simulink model "Galvo_sys_v20_scope"  (R2014a)
settings: Solver=ode45  StartTime=0.0  StopTime=5e-3  MaxStep=1e-4  RelTol=1e-3
InitFcn:
  | Kp_cc = evalin('base','Kp_cc');
  | init = evalin('base','init');
StartFcn:
  | Kp_cc = evalin('base','Kp_cc')
model workspace (MATLAB code in the model file):
  | Kp_cc = evalin('base','Kp_cc');
libraries: simulink x2
settings Model: Kp_cc=1  BufferReuse=off  Creator=mainster  LastModifiedBy=mainster
settings DataIOCC: SaveFormat=StructureWithTime
settings OptimizationCC: BlockReduction=off  InlineParams=on  OptimizeBlockIOStorage=off  BufferReuse=off  GlobalBufferReuse=off  ExpressionFolding=off  LocalBlockOutputs=off
settings DebuggingCC: UnderspecifiedInitializationDetection=Classic  StateNameClashWarn=warning  InitInArrayFormatMsg=none

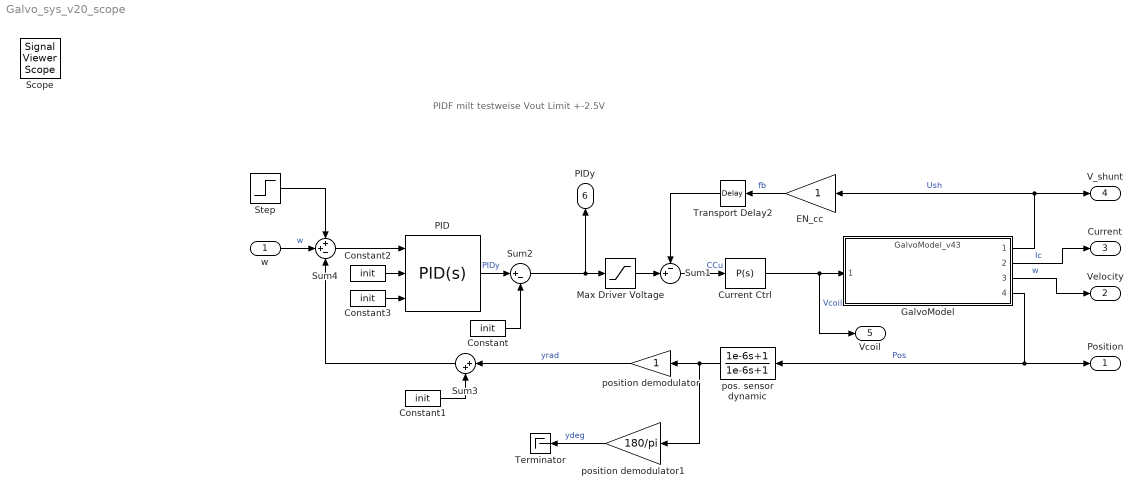
== system Galvo_sys_v20_scope ==
  note: PIDF milt testweise Vout Limit +-2.5V
  w : Inport
  Constant{,1..3} (4 alike) : Constant  Value=init
  Current Ctrl : simulink/Continuous/PID Controller  Controller=P  TimeDomain=Continuous-time  SampleTime=1  IntegratorMethod=Forward Euler  FilterMethod=Forward Euler  Form=Parallel  P=Kp_cc  I=1  D=0  N=100  InitialConditionSource=internal  InitialConditionForIntegrator=0  InitialConditionForFilter=0  ExternalReset=none  LimitOutput=off  UpperSaturationLimit=25  LowerSaturationLimit=-25  LinearizeAsGain=on  AntiWindupMode=none  Kb=1  TrackingMode=off  Kt=1  PParamMin=[]  PParamMax=[]  IParamMin=[]  IParamMax=[]  DParamMin=[]  DParamMax=[]  NParamMin=[]  NParamMax=[]  KbParamMin=[]  KbParamMax=[]  KtParamMin=[]  KtParamMax=[]  POutMin=[]  POutMax=[]  IOutMin=[]  IOutMax=[]  DOutMin=[]  DOutMax=[]  NOutMin=[]  NOutMax=[]  KbOutMin=[]  KbOutMax=[]  KtOutMin=[]  KtOutMax=[]  IntegratorOutMin=[]  IntegratorOutMax=[]  FilterOutMin=[]  FilterOutMax=[]  SumOutMin=[]  SumOutMax=[]  SumI1OutMin=[]  SumI1OutMax=[]  SumI2OutMin=[]  SumI2OutMax=[]  SumI3OutMin=[]  SumI3OutMax=[]  SumDOutMin=[]  SumDOutMax=[]  SaturationOutMin=[]  SaturationOutMax=[]  IntegratorContinuousStateAttributes=''  IntegratorStateMustResolveToSignalObject=off  IntegratorRTWStateStorageClass=Auto  FilterContinuousStateAttributes=''  FilterStateMustResolveToSignalObject=off  FilterRTWStateStorageClass=Auto
      settings: AttributesFormatString=Kp_cc=%<P>
  EN_cc : Gain
  GalvoModel : ModelReference  ModelNameDialog=GalvoModel_v43.slx  SimulationMode=Normal  Variant=on  OverrideUsingVariant=GalvoModel_v43  ModelReferenceVersion=1.49  CopyOfModelName=GalvoModel_v43.slx  DefaultDataLogging=on
      mask Display:
      | str=sprintf('%s',get(gcbh,'ModelName'));
      | port_label('input', 1, 'VCoil','texmode','on')
      | color('blue');
      | port_label('output', 1, 'VShunt','texmode','on')
      | color('black');
      | port_label('output', 2, 'Current')
      | port_label('output', 3, 'Velocity')
      | port_label('output', 4, 'Position')
      | %text(.05,.98,['{\fontsize{12}\it\bf' strrep(str,'_',' ') '}'],'horizontalAlignment','left','verticalAlignment','top','texmode','on')
      | text(.015,.98,['{\fontsize{12}\it\bf' strrep(str,'_','\_') '}'],'horizontalAlignment','left','verticalAlignment','top','texmode','on')
  Max Driver Voltage : Saturate  UpperLimit=25  LowerLimit=-25
      settings: AttributesFormatString=VoutMax=+-%<UpperLimit>
  PID : simulink/Continuous/PID Controller  Controller=PID  TimeDomain=Continuous-time  SampleTime=1  IntegratorMethod=Forward Euler  FilterMethod=Forward Euler  Form=Ideal  P=22.6304684101846  I=17.1701026929863  D=0.000767663019594148*1  N=7253.10376400166  InitialConditionSource=external  InitialConditionForIntegrator=1.25  InitialConditionForFilter=0  ExternalReset=none  IgnoreLimit=on  LimitOutput=on  UpperSaturationLimit=25  LowerSaturationLimit=-25  LinearizeAsGain=off  AntiWindupMode=back-calculation  Kb=6  TrackingMode=off  Kt=0  PParamMin=[]  PParamMax=[]  IParamMin=[]  IParamMax=[]  DParamMin=[]  DParamMax=[]  NParamMin=[]  NParamMax=[]  KbParamMin=[]  KbParamMax=[]  KtParamMin=[]  KtParamMax=[]  POutMin=[]  POutMax=[]  IOutMin=[]  IOutMax=[]  DOutMin=[]  DOutMax=[]  NOutMin=[]  NOutMax=[]  KbOutMin=[]  KbOutMax=[]  KtOutMin=[]  KtOutMax=[]  IntegratorOutMin=[]  IntegratorOutMax=[]  FilterOutMin=[]  FilterOutMax=[]  SumOutMin=[]  SumOutMax=[]  SumI1OutMin=[]  SumI1OutMax=[]  SumI2OutMin=[]  SumI2OutMax=[]  SumI3OutMin=[]  SumI3OutMax=[]  SumDOutMin=[]  SumDOutMax=[]  SaturationOutMin=[]  SaturationOutMax=[]  IntegratorContinuousStateAttributes=''  IntegratorStateMustResolveToSignalObject=off  IntegratorRTWStateStorageClass=Auto  FilterContinuousStateAttributes=''  FilterStateMustResolveToSignalObject=off  FilterRTWStateStorageClass=Auto
      settings: AttributesFormatString=AWM=%<AntiWindupMode>\nD=%<D>\nI=%<I>\nN=%<N>\nP=%<P>\nLimit=+-%<UpperSaturationLimit>
  Step : Step  Time=1e-3  After=0.2  SampleTime=0  ZeroCross=off
      settings: AttributesFormatString=Ampl.: %<After>
  Sum1 : Sum  Inputs=-+|
  Sum2 : Sum  Inputs=|+-
  Sum3 : Sum  Inputs=|++
  Sum4 : Sum  Inputs=++-
  Terminator : Terminator
  Transport Delay2 : TransportDelay  DelayTime=1e-9
      settings: AttributesFormatString=Delay=%<DelayTime>
  pos. sensor dynamic : TransferFcn  Numerator=[1e-6 1]  Denominator=[1e-6 1]
  position demodulator : Gain
  position demodulator1 : Gain  Gain=180/pi
  Position : Outport
  Velocity : Outport  Port=2
  Current : Outport  Port=3
  V_shunt : Outport  Port=4
  Vcoil : Outport  Port=5
  PIDy : Outport  Port=6
  Scope : SignalViewerScope  IOType=viewer  NumInputPorts=5  LegendLocations=|  RefreshTime=0.035000
      | 0.77344     0.92141     0.16354    0.025873
      | 0.78594     0.73642     0.15104    0.025873
      | 0.76094     0.55013     0.17604    0.025873
      | 0.79844     0.36384     0.13854    0.025873
      | 0.78594     0.17755     0.16354    0.046087
      settings: ShowLegends=on  TimeRange=0.005  YMin=-10~-0.5~-10~-5~-5  YMax=30~1~30~10~15
  wires:
  Sum4/1 -> PID/1
  Step/1 -> Sum4/1
  w/1 -> Sum4/2  "w"
  position demodulator/1 -> Sum3/1  "yrad"
  GalvoModel/1 -> V_shunt/1, EN_cc/1  "Ush"
  Sum1/1 -> Current Ctrl/1  "CCu"
  EN_cc/1 -> Transport Delay2/1  "fb"
  Transport Delay2/1 -> Sum1/1
  pos. sensor dynamic/1 -> position demodulator1/1, position demodulator/1
  GalvoModel/4 -> Position/1, pos. sensor dynamic/1  "Pos"
  GalvoModel/2 -> Current/1  "Ic"
  GalvoModel/3 -> Velocity/1  "w"
  Current Ctrl/1 -> GalvoModel/1, Vcoil/1  "Vcoil"
  Max Driver Voltage/1 -> Sum1/2
  PID/1 -> Sum2/1  "PIDy"
  Constant/1 -> Sum2/2
  Sum2/1 -> PIDy/1, Max Driver Voltage/1
  Sum3/1 -> Sum4/3
  Constant1/1 -> Sum3/2
  Constant2/1 -> PID/2
  Constant3/1 -> PID/3
  position demodulator1/1 -> Terminator/1  "ydeg"
